simulink model "quad_dynamics_sim_e"  (R2013a)
settings: Solver=ode3  StartTime=0.0  StopTime=30  FixedStep=0.01  RelTol=1e-3
values from neighbouring files (symbols this model uses):
  initial_states = [0;0;0;0;0;0;0.1;0;0.2;0;0.3;0]    [quad_dynamics_sim_script_e.m]
  params = [m;g;l;Jxx;Jyy;Jzz;k1;k2;k3;k4;b1;b2;b3;b4]    [quad_dynamics_sim_script_e.m]
  w = [w1; w2; w3; w4]    [quad_dynamics_sim_script_e.m]
settings Model: Creator=Ken Katagiri  LastModifiedBy=Ken Katagiri

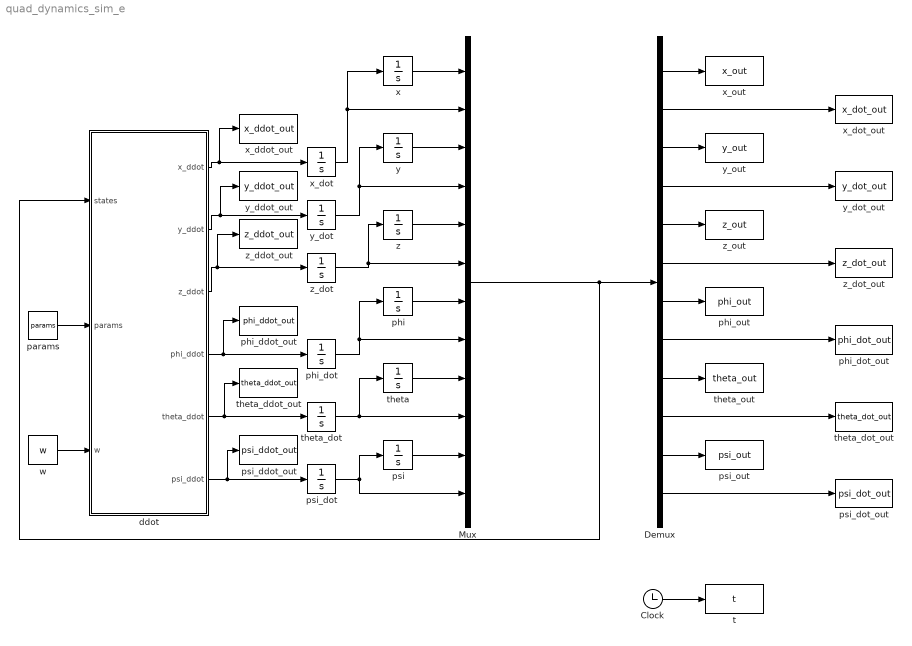
== system quad_dynamics_sim_e ==
  Clock : Clock
  Demux : Demux  Outputs=12
  Mux : Mux  Inputs=12
  ddot : MATLAB Function  TreatAsAtomicUnit=on
  params : Constant  Value=params
  phi : Integrator  InitialCondition=initial_states(7)
  phi_ddot_out : ToWorkspace  VariableName=phi_ddot_out  SampleTime=-1
  phi_dot : Integrator
  phi_dot_out : ToWorkspace  VariableName=phi_dot_out  SampleTime=-1
  phi_out : ToWorkspace  VariableName=phi_out  SampleTime=-1
  psi : Integrator  InitialCondition=initial_states(11)
  psi_ddot_out : ToWorkspace  VariableName=psi_ddot_out  SampleTime=-1
  psi_dot : Integrator
  psi_dot_out : ToWorkspace  VariableName=psi_dot_out  SampleTime=-1
  psi_out : ToWorkspace  VariableName=psi_out  SampleTime=-1
  t : ToWorkspace  VariableName=t  SampleTime=-1
  theta : Integrator  InitialCondition=initial_states(9)
  theta_ddot_out : ToWorkspace  VariableName=theta_ddot_out  SampleTime=-1
  theta_dot : Integrator
  theta_dot_out : ToWorkspace  VariableName=theta_dot_out  SampleTime=-1
  theta_out : ToWorkspace  VariableName=theta_out  SampleTime=-1
  w : Constant  Value=w
  x : Integrator  InitialCondition=initial_states(1)
  x_ddot_out : ToWorkspace  VariableName=x_ddot_out  SampleTime=-1
  x_dot : Integrator
  x_dot_out : ToWorkspace  VariableName=x_dot_out  SampleTime=-1
  x_out : ToWorkspace  VariableName=x_out  SampleTime=-1
  y : Integrator  InitialCondition=initial_states(3)
  y_ddot_out : ToWorkspace  VariableName=y_ddot_out  SampleTime=-1
  y_dot : Integrator
  y_dot_out : ToWorkspace  VariableName=y_dot_out  SampleTime=-1
  y_out : ToWorkspace  VariableName=y_out  SampleTime=-1
  z : Integrator  InitialCondition=initial_states(5)
  z_ddot_out : ToWorkspace  VariableName=z_ddot_out  SampleTime=-1
  z_dot : Integrator
  z_dot_out : ToWorkspace  VariableName=z_dot_out  SampleTime=-1
  z_out : ToWorkspace  VariableName=z_out  SampleTime=-1
  wires:
  ddot/1(x_ddot) -> x_ddot_out/1, x_dot/1
  ddot/2(y_ddot) -> y_ddot_out/1, y_dot/1
  ddot/3(z_ddot) -> z_ddot_out/1, z_dot/1
  x_dot/1 -> x/1, Mux/2
  y_dot/1 -> y/1, Mux/4
  psi_dot/1 -> psi/1, Mux/12
  theta_dot/1 -> Mux/10, theta/1
  phi_dot/1 -> Mux/8, phi/1
  x/1 -> Mux/1
  y/1 -> Mux/3
  z/1 -> Mux/5
  z_dot/1 -> z/1, Mux/6
  params/1 -> ddot/2(params)
  Clock/1 -> t/1
  Mux/1 -> ddot/1(states), Demux/1
  w/1 -> ddot/3(w)
  ddot/4(phi_ddot) -> phi_ddot_out/1, phi_dot/1
  ddot/5(theta_ddot) -> theta_ddot_out/1, theta_dot/1
  ddot/6(psi_ddot) -> psi_ddot_out/1, psi_dot/1
  phi/1 -> Mux/7
  theta/1 -> Mux/9
  psi/1 -> Mux/11
  Demux/1 -> x_out/1
  Demux/2 -> x_dot_out/1
  Demux/3 -> y_out/1
  Demux/4 -> y_dot_out/1
  Demux/5 -> z_out/1
  Demux/6 -> z_dot_out/1
  Demux/7 -> phi_out/1
  Demux/9 -> theta_out/1
  Demux/11 -> psi_out/1
  Demux/8 -> phi_dot_out/1
  Demux/10 -> theta_dot_out/1
  Demux/12 -> psi_dot_out/1

== matlab function quad_dynamics_sim_e/ddot ==
  data: states input size=12; x_ddot output; y_ddot output; z_ddot output; phi_ddot output; theta_ddot output; psi_ddot output; params input; w input
function [x_ddot, y_ddot, z_ddot, phi_ddot, theta_ddot, psi_ddot]= ddot(states, params, w)
%#codegen    
    m=params(1);
    g=params(2);
    l=params(3);

    Jxx=params(4);
    Jyy=params(5);
    Jzz=params(6);

    k1 = params(7);
    k2 = params(8);
    k3 = params(9);
    k4 = params(10);

    b1 = params(11);
    b2 = params(12);
    b3 = params(13);
    b4 = params(14);

    w1 = w(1);
    w2 = w(2);
    w3 = w(3);
    w4 = w(4);

    x = states(1); x_dot = states(2); y = states(3); y_dot = states(4); z = states(5); z_dot = states(6);
    phi = states(7); phi_dot = states(8); theta = states(9); theta_dot = states(10); psi = states(11); psi_dot = states(12);
        
        multipliers = ...
[Jxx*sin(psi)^2*sin(theta)^2+Jyy*cos(psi)^2*sin(theta)^2+Jzz*cos(theta)^2, Jxx*sin(psi)*sin(theta)*cos(psi)-Jyy*cos(psi)*sin(theta)*sin(psi), Jzz*cos(theta);
 Jxx*sin(psi)*sin(theta)*cos(psi)-Jyy*cos(psi)*sin(theta)*sin(psi), Jxx*cos(psi)^2+Jyy*sin(psi)^2, 0;
 Jzz*cos(theta), 0, Jzz];


    upphi_x = (k1*w1^2+k2*w2^2+k3*w3^2+k4*w4^2)*sin(theta)*sin(phi) ...
                + (-b1*w1^2+b2*w2^2+b3*w3^2-b4*w4^2)*(cos(psi)*cos(phi)-sin(psi)*cos(theta)*sin(phi)) ...
                + (b1*w1^2+b2*w2^2-b3*w3^2-b4*w4^2)*(-sin(psi)*cos(phi)-cos(psi)*cos(theta)*sin(phi));
            
    upphi_y = -(k1*w1^2+k2*w2^2+k3*w3^2+k4*w4^2)*sin(theta)*cos(phi) ...
                + (-b1*w1^2+b2*w2^2+b3*w3^2-b4*w4^2)*(cos(psi)*sin(phi)+sin(psi)*cos(theta)*cos(phi)) ...
                + (b1*w1^2+b2*w2^2-b3*w3^2-b4*w4^2)*(-sin(psi)*sin(phi)+cos(psi)*cos(theta)*cos(phi));
            
    upphi_z = (k1*w1^2+k2*w2^2+k3*w3^2+k4*w4^2)*cos(theta) ...
                + (-b1*w1^2+b2*w2^2+b3*w3^2-b4*w4^2)*sin(psi)*sin(theta) ...
                + (b1*w1^2+b2*w2^2-b3*w3^2-b4*w4^2)*cos(psi)*sin(theta);
            
    T_e2E = ...
        [cos(psi)*cos(phi)-sin(psi)*cos(theta)*sin(phi), -sin(psi)*cos(phi)-cos(psi)*cos(theta)*sin(phi), sin(theta)*sin(phi);
         cos(psi)*sin(phi)+sin(psi)*cos(theta)*cos(phi), -sin(psi)*sin(phi)+cos(psi)*cos(theta)*cos(phi), -sin(theta)*cos(phi);
         sin(psi)*sin(theta), cos(psi)*sin(theta), cos(theta)];
     
    force_mult_1 = [-b1*w1^2-b3*w3^2; b1*w1^2+b3*w3^2; k1*w1^2-k3*w3^2];
    force_mult_2 = [b2*w2^2+b4*w4^2; b2*w2^2+b4*w4^2; k2*w2^2-k4*w4^2];
    
    dx1_dphi = (l/sqrt(2)) * ...
                [sin(psi)*sin(phi)-cos(psi)*cos(theta)*cos(phi)-cos(psi)*sin(phi)-sin(psi)*cos(theta)*cos(phi); ...
                cos(psi)*cos(phi)-sin(psi)*cos(theta)*sin(phi)-sin(psi)*cos(phi)-cos(psi)*cos(theta)*sin(phi); ...
                0];
            
    dx2_dphi = (l/sqrt(2)) * ...
                [sin(psi)*sin(phi)-cos(psi)*cos(theta)*cos(phi)+cos(psi)*sin(phi)+sin(psi)*cos(theta)*cos(phi); ...
                -sin(psi)*cos(phi)-cos(psi)*cos(theta)*sin(phi)-cos(psi)*cos(phi)+sin(psi)*cos(theta)*sin(phi); ...
                0];
                
    upphi_phi = dot(T_e2E*force_mult_1, dx1_dphi) + dot(T_e2E*force_mult_2, dx2_dphi);
    
    
    dx1_dtheta = (l/sqrt(2)) * ...
                [sin(psi)*sin(theta)*sin(phi)+cos(psi)*sin(theta)*sin(phi);
                -sin(psi)*sin(theta)*cos(phi)-cos(psi)*sin(theta)*cos(phi);
                sin(psi)*cos(theta)+cos(psi)*cos(theta)];
    
    dx2_dtheta = (l/sqrt(2)) * ...
                [cos(psi)*sin(theta)*sin(phi)-sin(psi)*sin(theta)*sin(phi);
                -cos(psi)*sin(theta)*cos(phi)+sin(psi)*sin(theta)*cos(phi);
                cos(psi)*cos(theta)-sin(psi)*cos(theta)];

    upphi_theta = dot(T_e2E*force_mult_1, dx1_dtheta) + dot(T_e2E*force_mult_2, dx2_dtheta);
    
    
    dx1_dpsi = (l/sqrt(2)) * ...
                [-cos(phi)*sin(psi)-cos(theta)*sin(phi)*cos(psi)-cos(psi)*cos(phi)+sin(phi)*cos(theta)*sin(psi);
                -sin(phi)*sin(psi)+cos(theta)*cos(phi)*cos(psi)-sin(phi)*cos(psi)-cos(phi)*cos(theta)*sin(psi);
                sin(theta)*cos(psi)-sin(theta)*sin(psi)];
            
    dx2_dpsi = (l/sqrt(2)) * ...
                [-cos(psi)*cos(phi)+sin(phi)*cos(theta)*sin(psi)+cos(phi)*sin(psi)+cos(theta)*sin(phi)*cos(psi);
                -sin(phi)*cos(psi)-cos(phi)*cos(theta)*sin(psi)+sin(phi)*sin(psi)-cos(theta)*cos(phi)*cos(psi);
                -sin(theta)*sin(psi)-sin(theta)*cos(psi)];
            
    upphi_psi = dot(T_e2E*force_mult_1, dx1_dpsi) + dot(T_e2E*force_mult_2, dx2_dpsi);
    
    delta1 = upphi_phi ...
            -2*Jxx*sin(psi)^2*sin(theta)*cos(theta)*theta_dot*phi_dot - 2*Jxx*sin(psi)*cos(psi)*sin(theta)^2*psi_dot*phi_dot ...
            +Jxx*sin(psi)^2*sin(theta)*psi_dot*theta_dot - Jxx*sin(psi)*cos(theta)*cos(psi)*theta_dot^2 - Jxx*cos(psi)^2*sin(theta)*psi_dot*theta_dot ...
            -2*Jyy*sin(theta)*cos(theta)*cos(psi)^2*theta_dot*phi_dot + 2*Jyy*cos(psi)*sin(psi)*sin(theta)^2*psi_dot*phi_dot ...
            +Jyy*cos(psi)^2*sin(theta)*psi_dot*theta_dot + Jyy*cos(psi)*cos(theta)*sin(psi)*theta_dot^2 ...
            -Jyy*sin(psi)^2*sin(theta)*psi_dot*theta_dot + 2*Jzz*cos(theta)*sin(theta)*theta_dot*phi_dot + Jzz*sin(theta)*theta_dot*psi_dot;

    delta2 = upphi_theta ...
            + Jxx*sin(psi)^2*sin(theta)*psi_dot*phi_dot - Jxx*cos(psi)^2*sin(theta)*psi_dot*phi_dot ...
            + 2*Jxx*cos(psi)*sin(psi)*psi_dot*theta_dot + Jxx*sin(psi)^2*sin(theta)*cos(theta)*phi_dot^2 ...
            + Jyy*cos(psi)^2*sin(theta)*psi_dot*phi_dot - Jyy*sin(psi)^2*sin(theta)*psi_dot*phi_dot ...
            - 2*Jyy*sin(psi)*cos(psi)*psi_dot*theta_dot + Jyy*cos(psi)^2*sin(theta)*cos(theta)*phi_dot^2 ...
            - Jzz*sin(theta)*cos(theta)*phi_dot^2 - Jzz*sin(theta)*phi_dot*psi_dot;

    delta3 = upphi_psi ...
            + Jxx*sin(theta)^2*sin(psi)*cos(psi)*phi_dot^2 - Jxx*sin(theta)*sin(psi)^2*phi_dot*theta_dot ...
            + Jxx*sin(theta)*cos(psi)^2*phi_dot*theta_dot - Jxx*cos(psi)*sin(psi)*theta_dot^2 ...
            - Jyy*sin(theta)^2*cos(psi)*sin(psi)*phi_dot^2 - Jyy*sin(theta)*cos(psi)^2*phi_dot*theta_dot ...
            + Jyy*sin(theta)*sin(psi)^2*phi_dot*theta_dot + Jyy*sin(psi)*cos(psi)*theta_dot^2 + Jzz*sin(theta)*theta_dot*phi_dot;


    ddot = multipliers \ [delta1; delta2; delta3];


    x_ddot = upphi_x/m;
    y_ddot = upphi_y/m;
    z_ddot = upphi_z/m - g;
    phi_ddot = ddot(1);
    theta_ddot = ddot(2);
    psi_ddot = ddot(3);
